simulink model "PassStCshnFldIsPosChk"  (R2018b)
settings: Solver=FixedStepDiscrete  StartTime=0.0  StopTime=10.0  RelTol=1e-3
undefined symbols (not defined in the file or in its folder): KeSMSuFirstRwStCushFoldPosDelta_Val, KeSMSuFirstRwStCushFoldPosTolr_Val
libraries: StIsPosChkLib x7, simulink x5
settings Model: Creator=sn2xws  LastModifiedBy=sn2xws
settings Model: ModifiedHistory=|
  | 2024.6.26 V3.0.0 557模式流程
  | 2024.10.14 V3.0.1 新增模式Md57，Md58
  | 25.7.1 V3.13.0 新增Md61 Md62
settings DataIOCC: SaveFormat=StructureWithTime
settings OptimizationCC: DefaultParameterBehavior=Inlined  EnhancedBackFolding=on  PassReuseOutputArgsAs=Individual arguments  ZeroExternalMemoryAtStartup=off  ZeroInternalMemoryAtStartup=off  OptimizeBlockOrder=speed  DifferentSizesBufferReuse=on  OptimizationCustomize=off
settings DebuggingCC: ParameterTunabilityLossMsg=error
settings SFSimCC: MATLABDynamicMemAlloc=off
settings RTWCC: SystemTargetFile=autosar.tlc  GenCodeOnly=on  TemplateMakefile=ert_default_tmf  Description=AUTOSAR  GenerateReport=on  IncludeHyperlinkInReport=on  LaunchReport=on  GenerateTraceInfo=on  GenerateTraceReport=on  GenerateTraceReportSl=on  GenerateTraceReportSf=on  GenerateTraceReportEml=on
settings CodeAppCC: ForceParamTrailComments=on  IgnoreCustomStorageClasses=off  OperatorAnnotations=on  SimulinkDataObjDesc=on  SFDataObjDesc=on  InsertBlockDesc=on
settings STFCustomTargetCC: TargetLangStandard=C99 (ISO)  MultiwordLength=256  ParMdlRefBuildCompliant=on  CompOptLevelCompliant=on  IncludeMdlTerminateFcn=off  CombineOutputUpdateFcns=on  SuppressErrorStatus=on  ERTCustomFileBanners=on  SupportNonFinite=off  SupportComplex=off  SupportContinuousTime=off  SupportNonInlinedSFcns=off  RemoveResetFunc=on  MATLABClassNameForMDSCustomization=Simulink.SoftwareTarget.ERTCustomization  AutosarCompliant=on  UseToolchainInfoCompliant=on  LookupTableObjectStructAxisOrder=2,1,3,4,...  LUTObjectStructOrderEvenSpacing=Size,Table,Breakpoints  SystemTargetFile=autosar.tlc
settings ERTTargetCC: TargetLangStandard=C99 (ISO)  ConcurrentExecutionCompliant=off  IncludeMdlTerminateFcn=off  SuppressErrorStatus=on  SupportNonFinite=off  SupportComplex=off  ModelStepFunctionPrototypeControlCompliant=off  CPPClassGenCompliant=off  AutosarCompliant=on  LookupTableObjectStructAxisOrder=2,1,3,4,...  LUTObjectStructOrderEvenSpacing=Size,Table,Breakpoints  InlinedParameterPlacement=NonHierarchical  ERTCustomFileTemplate=example_file_process.tlc  ERTFilePackagingFormat=Compact

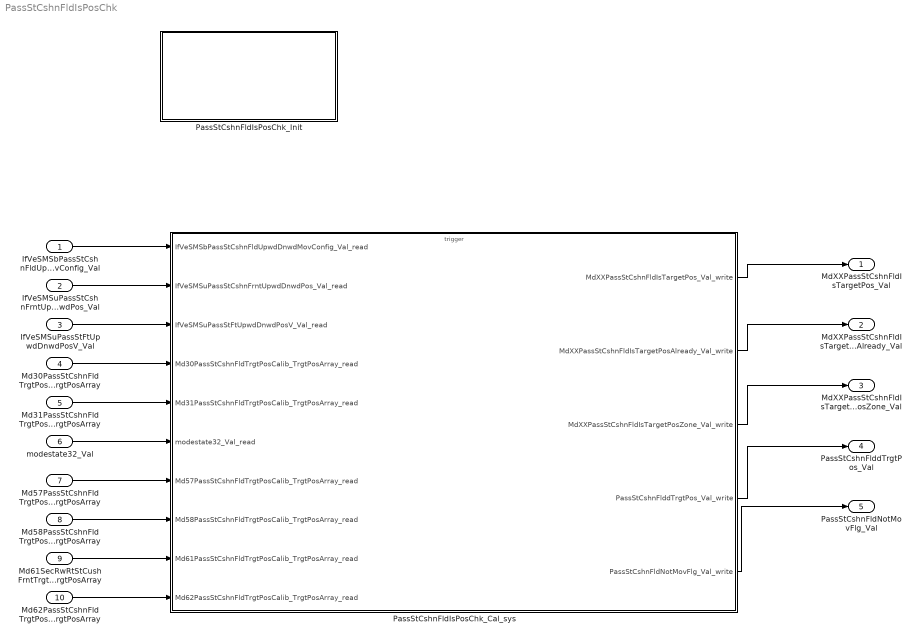
== system PassStCshnFldIsPosChk ==
  IfVeSMSbPassStCshnFldUpwdDnwdMovConfig_Val : Inport  OutDataTypeStr=boolean  PortDimensions=1
  IfVeSMSuPassStCshnFrntUpwdDnwdPos_Val : Inport  Port=2  OutDataTypeStr=uint16  PortDimensions=1
  IfVeSMSuPassStFtUpwdDnwdPosV_Val : Inport  Port=3  OutDataTypeStr=boolean  PortDimensions=1
  Md30PassStCshnFldTrgtPosCalib_TrgtPosArray : Inport  Description=|  Port=4  OutDataTypeStr=uint16  PortDimensions=3
      | 0:Pos
      | 1:Max
      | 2:Min
  Md31PassStCshnFldTrgtPosCalib_TrgtPosArray : Inport  Description=|  Port=5  OutDataTypeStr=uint16  PortDimensions=3
      | 0:Pos
      | 1:Max
      | 2:Min
  modestate32_Val : Inport  Port=6  OutDataTypeStr=uint32  PortDimensions=1
  Md57PassStCshnFldTrgtPosCalib_TrgtPosArray : Inport  Description=|  Port=7  OutDataTypeStr=uint16  PortDimensions=3
      | 0:Pos
      | 1:Max
      | 2:Min
  Md58PassStCshnFldTrgtPosCalib_TrgtPosArray : Inport  Description=|  Port=8  OutDataTypeStr=uint16  PortDimensions=3
      | 0:Pos
      | 1:Max
      | 2:Min
  Md61SecRwRtStCushFrntTrgtPosCalib_TrgtPosArray : Inport  Description=|  Port=9  OutDataTypeStr=uint16  PortDimensions=3
      | 0:Pos
      | 1:Max
      | 2:Min
  Md62PassStCshnFldTrgtPosCalib_TrgtPosArray : Inport  Description=|  Port=10  OutDataTypeStr=uint16  PortDimensions=3
      | 0:Pos
      | 1:Max
      | 2:Min
  PassStCshnFldIsPosChk_Cal_sys : Subsystem
  PassStCshnFldIsPosChk_Init : Subsystem
  MdXXPassStCshnFldIsTargetPos_Val : Outport  OutDataTypeStr=uint32  PortDimensions=1
  MdXXPassStCshnFldIsTargetPosAlready_Val : Outport  Port=2  OutDataTypeStr=uint32  PortDimensions=1
  MdXXPassStCshnFldIsTargetPosZone_Val : Outport  Port=3  OutDataTypeStr=uint32  PortDimensions=1
  PassStCshnFlddTrgtPos_Val : Outport  Port=4  OutDataTypeStr=uint16  PortDimensions=1
  PassStCshnFldNotMovFlg_Val : Outport  Port=5  OutDataTypeStr=boolean  PortDimensions=1
  wires:
  IfVeSMSbPassStCshnFldUpwdDnwdMovConfig_Val/1 -> PassStCshnFldIsPosChk_Cal_sys/1(IfVeSMSbPassStCshnFldUpwdDnwdMovConfig_Val_read)
  IfVeSMSuPassStCshnFrntUpwdDnwdPos_Val/1 -> PassStCshnFldIsPosChk_Cal_sys/2(IfVeSMSuPassStCshnFrntUpwdDnwdPos_Val_read)
  IfVeSMSuPassStFtUpwdDnwdPosV_Val/1 -> PassStCshnFldIsPosChk_Cal_sys/3(IfVeSMSuPassStFtUpwdDnwdPosV_Val_read)
  Md30PassStCshnFldTrgtPosCalib_TrgtPosArray/1 -> PassStCshnFldIsPosChk_Cal_sys/4(Md30PassStCshnFldTrgtPosCalib_TrgtPosArray_read)
  Md31PassStCshnFldTrgtPosCalib_TrgtPosArray/1 -> PassStCshnFldIsPosChk_Cal_sys/5(Md31PassStCshnFldTrgtPosCalib_TrgtPosArray_read)
  modestate32_Val/1 -> PassStCshnFldIsPosChk_Cal_sys/6(modestate32_Val_read)
  PassStCshnFldIsPosChk_Cal_sys/1(MdXXPassStCshnFldIsTargetPos_Val_write) -> MdXXPassStCshnFldIsTargetPos_Val/1
  PassStCshnFldIsPosChk_Cal_sys/2(MdXXPassStCshnFldIsTargetPosAlready_Val_write) -> MdXXPassStCshnFldIsTargetPosAlready_Val/1
  PassStCshnFldIsPosChk_Cal_sys/3(MdXXPassStCshnFldIsTargetPosZone_Val_write) -> MdXXPassStCshnFldIsTargetPosZone_Val/1
  PassStCshnFldIsPosChk_Cal_sys/4(PassStCshnFlddTrgtPos_Val_write) -> PassStCshnFlddTrgtPos_Val/1
  PassStCshnFldIsPosChk_Cal_sys/5(PassStCshnFldNotMovFlg_Val_write) -> PassStCshnFldNotMovFlg_Val/1
  Md57PassStCshnFldTrgtPosCalib_TrgtPosArray/1 -> PassStCshnFldIsPosChk_Cal_sys/7(Md57PassStCshnFldTrgtPosCalib_TrgtPosArray_read)
  Md58PassStCshnFldTrgtPosCalib_TrgtPosArray/1 -> PassStCshnFldIsPosChk_Cal_sys/8(Md58PassStCshnFldTrgtPosCalib_TrgtPosArray_read)
  Md61SecRwRtStCushFrntTrgtPosCalib_TrgtPosArray/1 -> PassStCshnFldIsPosChk_Cal_sys/9(Md61PassStCshnFldTrgtPosCalib_TrgtPosArray_read)
  Md62PassStCshnFldTrgtPosCalib_TrgtPosArray/1 -> PassStCshnFldIsPosChk_Cal_sys/10(Md62PassStCshnFldTrgtPosCalib_TrgtPosArray_read)

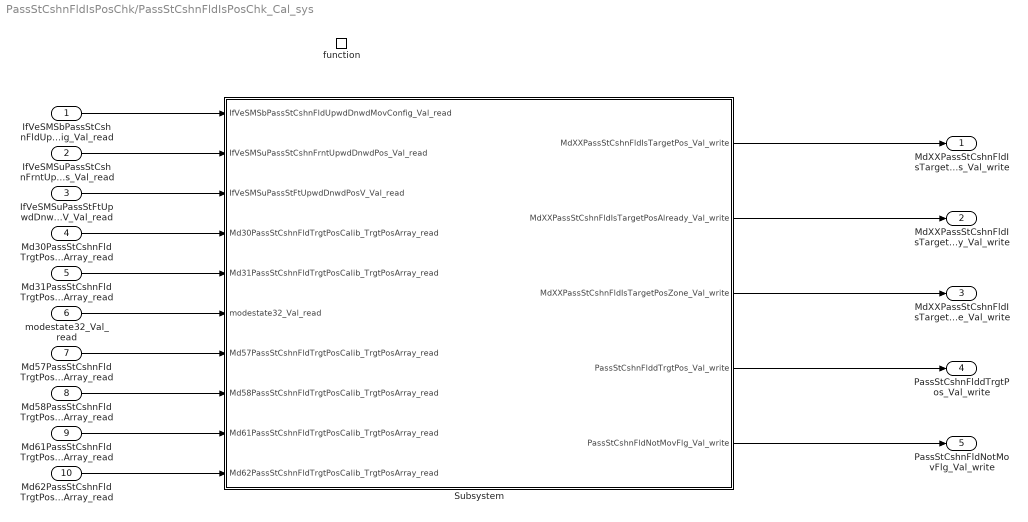
== system PassStCshnFldIsPosChk/PassStCshnFldIsPosChk_Cal_sys ==
  IfVeSMSbPassStCshnFldUpwdDnwdMovConfig_Val_read : Inport
  IfVeSMSuPassStCshnFrntUpwdDnwdPos_Val_read : Inport  Port=2
  IfVeSMSuPassStFtUpwdDnwdPosV_Val_read : Inport  Port=3
  Md30PassStCshnFldTrgtPosCalib_TrgtPosArray_read : Inport  Port=4
  Md31PassStCshnFldTrgtPosCalib_TrgtPosArray_read : Inport  Port=5
  modestate32_Val_read : Inport  Port=6
  Md57PassStCshnFldTrgtPosCalib_TrgtPosArray_read : Inport  Port=7
  Md58PassStCshnFldTrgtPosCalib_TrgtPosArray_read : Inport  Port=8
  Md61PassStCshnFldTrgtPosCalib_TrgtPosArray_read : Inport  Port=9
  Md62PassStCshnFldTrgtPosCalib_TrgtPosArray_read : Inport  Port=10
  function : TriggerPort  TriggerType=function-call  IsSimulinkFunction=on  FunctionName=PassStCshnFldIsPosChk_Cal  VariantControl=(inherit)
  Subsystem : Subsystem
  MdXXPassStCshnFldIsTargetPos_Val_write : Outport
      settings: EnsureOutportIsVirtual=on
  MdXXPassStCshnFldIsTargetPosAlready_Val_write : Outport  Port=2
      settings: EnsureOutportIsVirtual=on
  MdXXPassStCshnFldIsTargetPosZone_Val_write : Outport  Port=3
      settings: EnsureOutportIsVirtual=on
  PassStCshnFlddTrgtPos_Val_write : Outport  Port=4
      settings: EnsureOutportIsVirtual=on
  PassStCshnFldNotMovFlg_Val_write : Outport  Port=5
      settings: EnsureOutportIsVirtual=on
  wires:
  IfVeSMSbPassStCshnFldUpwdDnwdMovConfig_Val_read/1 -> Subsystem/1(IfVeSMSbPassStCshnFldUpwdDnwdMovConfig_Val_read)
  IfVeSMSuPassStCshnFrntUpwdDnwdPos_Val_read/1 -> Subsystem/2(IfVeSMSuPassStCshnFrntUpwdDnwdPos_Val_read)
  IfVeSMSuPassStFtUpwdDnwdPosV_Val_read/1 -> Subsystem/3(IfVeSMSuPassStFtUpwdDnwdPosV_Val_read)
  Md30PassStCshnFldTrgtPosCalib_TrgtPosArray_read/1 -> Subsystem/4(Md30PassStCshnFldTrgtPosCalib_TrgtPosArray_read)
  Md31PassStCshnFldTrgtPosCalib_TrgtPosArray_read/1 -> Subsystem/5(Md31PassStCshnFldTrgtPosCalib_TrgtPosArray_read)
  modestate32_Val_read/1 -> Subsystem/6(modestate32_Val_read)
  Subsystem/1(MdXXPassStCshnFldIsTargetPos_Val_write) -> MdXXPassStCshnFldIsTargetPos_Val_write/1
  Subsystem/2(MdXXPassStCshnFldIsTargetPosAlready_Val_write) -> MdXXPassStCshnFldIsTargetPosAlready_Val_write/1
  Subsystem/3(MdXXPassStCshnFldIsTargetPosZone_Val_write) -> MdXXPassStCshnFldIsTargetPosZone_Val_write/1
  Subsystem/4(PassStCshnFlddTrgtPos_Val_write) -> PassStCshnFlddTrgtPos_Val_write/1
  Subsystem/5(PassStCshnFldNotMovFlg_Val_write) -> PassStCshnFldNotMovFlg_Val_write/1
  Md57PassStCshnFldTrgtPosCalib_TrgtPosArray_read/1 -> Subsystem/7(Md57PassStCshnFldTrgtPosCalib_TrgtPosArray_read)
  Md58PassStCshnFldTrgtPosCalib_TrgtPosArray_read/1 -> Subsystem/8(Md58PassStCshnFldTrgtPosCalib_TrgtPosArray_read)
  Md61PassStCshnFldTrgtPosCalib_TrgtPosArray_read/1 -> Subsystem/9(Md61PassStCshnFldTrgtPosCalib_TrgtPosArray_read)
  Md62PassStCshnFldTrgtPosCalib_TrgtPosArray_read/1 -> Subsystem/10(Md62PassStCshnFldTrgtPosCalib_TrgtPosArray_read)

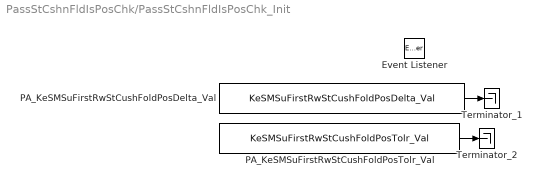
== system PassStCshnFldIsPosChk/PassStCshnFldIsPosChk_Init ==
  Event Listener : EventListener  EventName=reset
  PA_KeSMSuFirstRwStCushFoldPosDelta_Val : Constant  Value=KeSMSuFirstRwStCushFoldPosDelta_Val
  PA_KeSMSuFirstRwStCushFoldPosTolr_Val : Constant  Value=KeSMSuFirstRwStCushFoldPosTolr_Val
  Terminator_1 : Terminator
  Terminator_2 : Terminator
  wires:
  PA_KeSMSuFirstRwStCushFoldPosDelta_Val/1 -> Terminator_1/1
  PA_KeSMSuFirstRwStCushFoldPosTolr_Val/1 -> Terminator_2/1

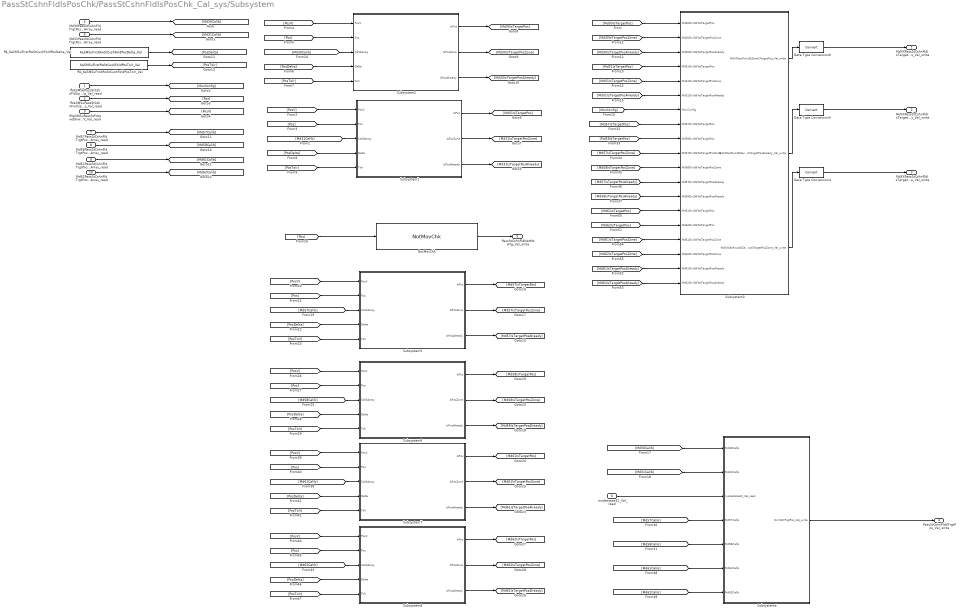
== system PassStCshnFldIsPosChk/PassStCshnFldIsPosChk_Cal_sys/Subsystem ==
  IfVeSMSbPassStCshnFldUpwdDnwdMovConfig_Val_read : Inport
  IfVeSMSuPassStCshnFrntUpwdDnwdPos_Val_read : Inport  Port=2
  IfVeSMSuPassStFtUpwdDnwdPosV_Val_read : Inport  Port=3
  Md30PassStCshnFldTrgtPosCalib_TrgtPosArray_read : Inport  Port=4
  Md31PassStCshnFldTrgtPosCalib_TrgtPosArray_read : Inport  Port=5
  modestate32_Val_read : Inport  Port=6
  Md57PassStCshnFldTrgtPosCalib_TrgtPosArray_read : Inport  Port=7
  Md58PassStCshnFldTrgtPosCalib_TrgtPosArray_read : Inport  Port=8
  Md61PassStCshnFldTrgtPosCalib_TrgtPosArray_read : Inport  Port=9
  Md62PassStCshnFldTrgtPosCalib_TrgtPosArray_read : Inport  Port=10
  Data Type Conversion4 : DataTypeConversion
  Data Type Conversion5 : DataTypeConversion
  Data Type Conversion6 : DataTypeConversion
  NotMovChk : StIsPosChkLib/NotMovChk  SystemSampleTime=-1
  PA_KeSMSuFirstRwStCushFoldPosDelta_Val : Constant  Value=KeSMSuFirstRwStCushFoldPosDelta_Val
  PA_KeSMSuFirstRwStCushFoldPosTolr_Val : Constant  Value=KeSMSuFirstRwStCushFoldPosTolr_Val
  Subsystem1 : Subsystem
  Subsystem2 : Subsystem
  Subsystem3 : Subsystem
  Subsystem4 : Subsystem
  Subsystem5 : Subsystem
  Subsystem6 : Subsystem
  Subsystem7 : Subsystem
  Subsystem8 : Subsystem
  MdXXPassStCshnFldIsTargetPos_Val_write : Outport
      settings: EnsureOutportIsVirtual=on
  MdXXPassStCshnFldIsTargetPosAlready_Val_write : Outport  Port=2
      settings: EnsureOutportIsVirtual=on
  MdXXPassStCshnFldIsTargetPosZone_Val_write : Outport  Port=3
      settings: EnsureOutportIsVirtual=on
  PassStCshnFlddTrgtPos_Val_write : Outport  Port=4
      settings: EnsureOutportIsVirtual=on
  PassStCshnFldNotMovFlg_Val_write : Outport  Port=5
      settings: EnsureOutportIsVirtual=on
  wires:
  modestate32_Val_read/1 -> Subsystem4/3(modestate32_Val_read)
  PA_KeSMSuFirstRwStCushFoldPosDelta_Val/1 -> [PosDelta]
  Md30PassStCshnFldTrgtPosCalib_TrgtPosArray_read/1 -> [Md30Calib]
  Md31PassStCshnFldTrgtPosCalib_TrgtPosArray_read/1 -> [Md31Calib]
  IfVeSMSbPassStCshnFldUpwdDnwdMovConfig_Val_read/1 -> [MovConfig]
  IfVeSMSuPassStCshnFrntUpwdDnwdPos_Val_read/1 -> [Pos]
  IfVeSMSuPassStFtUpwdDnwdPosV_Val_read/1 -> [PosV]
  PA_KeSMSuFirstRwStCushFoldPosTolr_Val/1 -> [PosTolr]
  Data Type Conversion4/1 -> MdXXPassStCshnFldIsTargetPosZone_Val_write/1
  Data Type Conversion6/1 -> MdXXPassStCshnFldIsTargetPos_Val_write/1
  Subsystem3/3(MdXXSecRwLtStZeroIsTargetPosZone_Val_write) -> Data Type Conversion4/1
  Subsystem3/2(MdXXSecRwLtStZeroIsTargetPosAlready_Val_write) -> Data Type Conversion5/1
  [MovConfig] -> Subsystem3/7(MovConfig)
  [Md30IsTargetPosAlready] -> Subsystem3/3(Md30DrvStFtIsTargetPosAlready)
  Data Type Conversion5/1 -> MdXXPassStCshnFldIsTargetPosAlready_Val_write/1
  [PosTolr] -> Subsystem1/5(Tolr)
  [Md31Calib] -> Subsystem1/3(CalibArray)
  Subsystem1/3(IsPosAlready) -> [Md31IsTargetPosAlready]
  [PosDelta] -> Subsystem1/4(Delta)
  [Pos] -> Subsystem1/2(Pos)
  [PosV] -> Subsystem1/1(PosV)
  Subsystem1/1(IsPos) -> [Md31IsTargetPos]
  Subsystem1/2(IsPosZone) -> [Md31IsTargetPosZone]
  [PosTolr] -> Subsystem2/5(Tolr)
  [PosV] -> Subsystem2/1(PosV)
  Subsystem2/2(IsPosZone) -> [Md30IsTargetPosZone]
  [Md30IsTargetPos] -> Subsystem3/1(Md30DrvStFtIsTargetPos)
  [Md31IsTargetPosZone] -> Subsystem3/5(Md31DrvStFtIsTargetPosZone)
  Subsystem2/1(IsPos) -> [Md30IsTargetPos]
  [Pos] -> Subsystem2/2(Pos)
  [Md31IsTargetPosAlready] -> Subsystem3/6(Md31DrvStFtIsTargetPosAlready)
  [PosDelta] -> Subsystem2/4(Delta)
  [Md30Calib] -> Subsystem2/3(CalibArray)
  Subsystem3/1(MdXXSecRwLtStZeroIsTargetPos_Val_write) -> Data Type Conversion6/1
  Subsystem2/3(IsPosAlready) -> [Md30IsTargetPosAlready]
  [Md31IsTargetPos] -> Subsystem3/4(Md31DrvStFtIsTargetPos)
  [Md30IsTargetPosZone] -> Subsystem3/2(Md30DrvStFtIsTargetPosZone)
  NotMovChk/1 -> PassStCshnFldNotMovFlg_Val_write/1
  [Pos] -> NotMovChk/1
  [Md31Calib] -> Subsystem4/2(Md31Calib)
  Subsystem4/1(DrvStFtTrgtPos_Val_write) -> PassStCshnFlddTrgtPos_Val_write/1
  [Md30Calib] -> Subsystem4/1(Md30Calib)
  Md57PassStCshnFldTrgtPosCalib_TrgtPosArray_read/1 -> [Md57Calib]
  Md58PassStCshnFldTrgtPosCalib_TrgtPosArray_read/1 -> [Md58Calib]
  Subsystem5/2(IsPosZone) -> [Md57IsTargetPosZone]
  Subsystem5/1(IsPos) -> [Md57IsTargetPos]
  [PosV] -> Subsystem5/1(PosV)
  [Pos] -> Subsystem5/2(Pos)
  [PosDelta] -> Subsystem5/4(Delta)
  Subsystem5/3(IsPosAlready) -> [Md57IsTargetPosAlready]
  [Md57Calib] -> Subsystem5/3(CalibArray)
  [PosTolr] -> Subsystem5/5(Tolr)
  [PosTolr] -> Subsystem6/5(Tolr)
  [Md58Calib] -> Subsystem6/3(CalibArray)
  Subsystem6/3(IsPosAlready) -> [Md58IsTargetPosAlready]
  [PosDelta] -> Subsystem6/4(Delta)
  [Pos] -> Subsystem6/2(Pos)
  [PosV] -> Subsystem6/1(PosV)
  Subsystem6/1(IsPos) -> [Md58IsTargetPos]
  Subsystem6/2(IsPosZone) -> [Md58IsTargetPosZone]
  [Md57Calib] -> Subsystem4/4(Md57Calib)
  [Md58Calib] -> Subsystem4/5(Md58Calib)
  [Md57IsTargetPos] -> Subsystem3/8(Md57DrvStFtIsTargetPos)
  [Md58IsTargetPos] -> Subsystem3/9(Md58DrvStFtIsTargetPos)
  [Md57IsTargetPosZone] -> Subsystem3/10(Md57DrvStFtIsTargetPosZone)
  [Md58IsTargetPosZone] -> Subsystem3/11(Md58DrvStFtIsTargetPosZone)
  [Md58IsTargetPosAlready] -> Subsystem3/13(Md58DrvStFtIsTargetPosAlready)
  [Md57IsTargetPosAlready] -> Subsystem3/12(Md57DrvStFtIsTargetPosAlready)
  Md61PassStCshnFldTrgtPosCalib_TrgtPosArray_read/1 -> [Md61Calib]
  Md62PassStCshnFldTrgtPosCalib_TrgtPosArray_read/1 -> [Md62Calib]
  Subsystem7/2(IsPosZone) -> [Md61IsTargetPosZone]
  Subsystem7/1(IsPos) -> [Md61IsTargetPos]
  [PosV] -> Subsystem7/1(PosV)
  [Pos] -> Subsystem7/2(Pos)
  [PosDelta] -> Subsystem7/4(Delta)
  Subsystem7/3(IsPosAlready) -> [Md61IsTargetPosAlready]
  [Md61Calib] -> Subsystem7/3(CalibArray)
  [PosTolr] -> Subsystem7/5(Tolr)
  [PosTolr] -> Subsystem8/5(Tolr)
  [Md62Calib] -> Subsystem8/3(CalibArray)
  Subsystem8/3(IsPosAlready) -> [Md62IsTargetPosAlready]
  [PosDelta] -> Subsystem8/4(Delta)
  [Pos] -> Subsystem8/2(Pos)
  [PosV] -> Subsystem8/1(PosV)
  Subsystem8/1(IsPos) -> [Md62IsTargetPos]
  Subsystem8/2(IsPosZone) -> [Md62IsTargetPosZone]
  [Md61Calib] -> Subsystem4/6(Md61Calib)
  [Md62Calib] -> Subsystem4/7(Md62Calib)
  [Md61IsTargetPos] -> Subsystem3/14(Md61DrvStFtIsTargetPos)
  [Md62IsTargetPos] -> Subsystem3/15(Md62DrvStFtIsTargetPos)
  [Md61IsTargetPosZone] -> Subsystem3/16(Md61DrvStFtIsTargetPosZone)
  [Md62IsTargetPosZone] -> Subsystem3/17(Md62DrvStFtIsTargetPosZone)
  [Md61IsTargetPosAlready] -> Subsystem3/18(Md61DrvStFtIsTargetPosAlready)
  [Md62IsTargetPosAlready] -> Subsystem3/19(Md62DrvStFtIsTargetPosAlready)

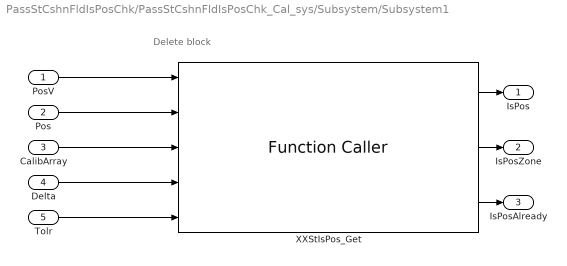
== system PassStCshnFldIsPosChk/PassStCshnFldIsPosChk_Cal_sys/Subsystem/Subsystem1 ==
  note: Delete block
  PosV : Inport
  Pos : Inport  Port=2
  CalibArray : Inport  Port=3
  Delta : Inport  Port=4
  Tolr : Inport  Port=5
  XXStIsPos_Get : FunctionCaller  FunctionPrototype=[IsPos,IsPosZone,IsPosAlready] = XXStIsPos_Get(PosV,Pos,CalibArray,Delta,Tolr)  InputArgumentSpecifications=boolean(true), uint16(1), uint16([1;1;1]), uint16(1), uint16(1)  OutputArgumentSpecifications=boolean(true), boolean(true), boolean(true)
  IsPos : Outport
  IsPosZone : Outport  Port=2
  IsPosAlready : Outport  Port=3
  wires:
  Delta/1 -> XXStIsPos_Get/4
  Tolr/1 -> XXStIsPos_Get/5
  PosV/1 -> XXStIsPos_Get/1
  XXStIsPos_Get/2 -> IsPosZone/1
  Pos/1 -> XXStIsPos_Get/2
  XXStIsPos_Get/1 -> IsPos/1
  CalibArray/1 -> XXStIsPos_Get/3
  XXStIsPos_Get/3 -> IsPosAlready/1

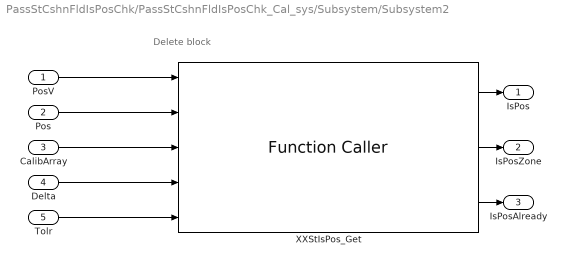
== system PassStCshnFldIsPosChk/PassStCshnFldIsPosChk_Cal_sys/Subsystem/Subsystem2 ==
  note: Delete block
  PosV : Inport
  Pos : Inport  Port=2
  CalibArray : Inport  Port=3
  Delta : Inport  Port=4
  Tolr : Inport  Port=5
  XXStIsPos_Get : FunctionCaller  FunctionPrototype=[IsPos,IsPosZone,IsPosAlready] = XXStIsPos_Get(PosV,Pos,CalibArray,Delta,Tolr)  InputArgumentSpecifications=boolean(true), uint16(1), uint16([1;1;1]), uint16(1), uint16(1)  OutputArgumentSpecifications=boolean(true), boolean(true), boolean(true)
  IsPos : Outport
  IsPosZone : Outport  Port=2
  IsPosAlready : Outport  Port=3
  wires:
  XXStIsPos_Get/3 -> IsPosAlready/1
  CalibArray/1 -> XXStIsPos_Get/3
  XXStIsPos_Get/1 -> IsPos/1
  Pos/1 -> XXStIsPos_Get/2
  XXStIsPos_Get/2 -> IsPosZone/1
  PosV/1 -> XXStIsPos_Get/1
  Tolr/1 -> XXStIsPos_Get/5
  Delta/1 -> XXStIsPos_Get/4

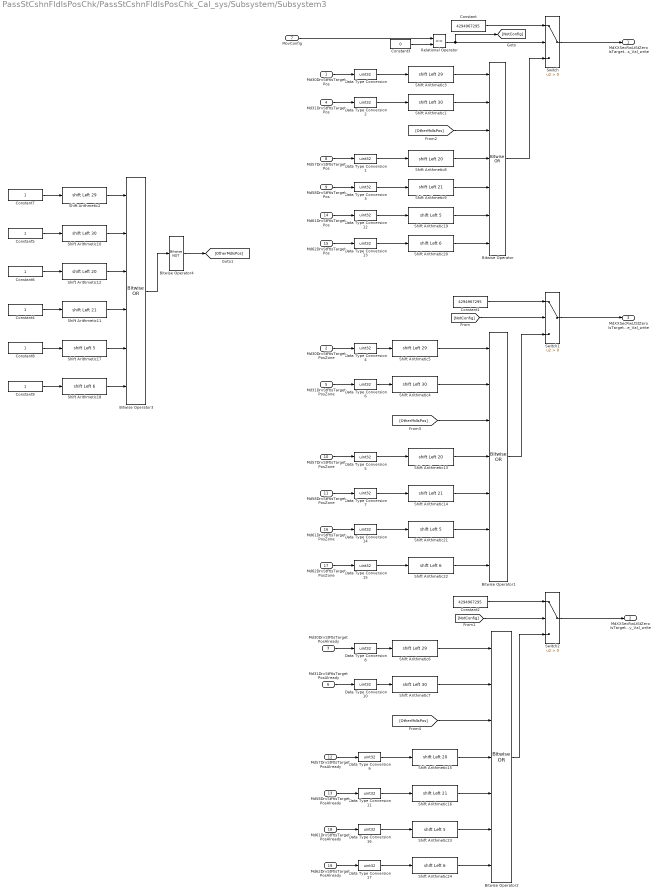
== system PassStCshnFldIsPosChk/PassStCshnFldIsPosChk_Cal_sys/Subsystem/Subsystem3 ==
  Md30DrvStFtIsTargetPos : Inport
  Md30DrvStFtIsTargetPosZone : Inport  Port=2
  Md30DrvStFtIsTargetPosAlready : Inport  Port=3
  Md31DrvStFtIsTargetPos : Inport  Port=4
  Md31DrvStFtIsTargetPosZone : Inport  Port=5
  Md31DrvStFtIsTargetPosAlready : Inport  Port=6
  MovConfig : Inport  Port=7
  Md57DrvStFtIsTargetPos : Inport  Port=8
  Md58DrvStFtIsTargetPos : Inport  Port=9
  Md57DrvStFtIsTargetPosZone : Inport  Port=10
  Md58DrvStFtIsTargetPosZone : Inport  Port=11
  Md57DrvStFtIsTargetPosAlready : Inport  Port=12
  Md58DrvStFtIsTargetPosAlready : Inport  Port=13
  Md61DrvStFtIsTargetPos : Inport  Port=14
  Md62DrvStFtIsTargetPos : Inport  Port=15
  Md61DrvStFtIsTargetPosZone : Inport  Port=16
  Md62DrvStFtIsTargetPosZone : Inport  Port=17
  Md61DrvStFtIsTargetPosAlready : Inport  Port=18
  Md62DrvStFtIsTargetPosAlready : Inport  Port=19
  Bitwise Operator : simulink/Logic and Bit Operations/Bitwise Operator  logicop=OR  UseBitMask=off  NumInputPorts=7  BitMask=bin2dec('11011001')  BitMaskRealWorld=Stored Integer
  Bitwise Operator1 : simulink/Logic and Bit Operations/Bitwise Operator  logicop=OR  UseBitMask=off  NumInputPorts=7  BitMask=bin2dec('11011001')  BitMaskRealWorld=Stored Integer
  Bitwise Operator2 : simulink/Logic and Bit Operations/Bitwise Operator  logicop=OR  UseBitMask=off  NumInputPorts=7  BitMask=bin2dec('11011001')  BitMaskRealWorld=Stored Integer
  Bitwise Operator3 : simulink/Logic and Bit Operations/Bitwise Operator  logicop=OR  UseBitMask=off  NumInputPorts=6  BitMask=bin2dec('11011001')  BitMaskRealWorld=Stored Integer
  Bitwise Operator4 : simulink/Logic and Bit Operations/Bitwise Operator  logicop=NOT  UseBitMask=off  BitMask=bin2dec('11011001')  BitMaskRealWorld=Stored Integer
  Constant : Constant  Value=4294967295  OutDataTypeStr=uint32
  Constant1 : Constant  Value=4294967295  OutDataTypeStr=uint32
  Constant2 : Constant  Value=4294967295  OutDataTypeStr=uint32
  Constant3 : Constant  Value=0  OutDataTypeStr=uint8
  Constant{4..9} (6 alike) : Constant  OutDataTypeStr=uint32
  Data Type Conversion{,1..17} (18 alike) : DataTypeConversion  OutDataTypeStr=uint32
  Relational Operator : RelationalOperator  Operator===  OutDataTypeStr=boolean  RndMeth=Simplest
  Shift Arithmetic{1,4,7,10} (4 alike) : ArithShift  BitShiftNumber=30  BitShiftDirection=Left
  Shift Arithmetic{9,11,14,16} (4 alike) : ArithShift  BitShiftNumber=21  BitShiftDirection=Left
  Shift Arithmetic{8,12..13,15} (4 alike) : ArithShift  BitShiftNumber=20  BitShiftDirection=Left
  Shift Arithmetic{17,19,21,23} (4 alike) : ArithShift  BitShiftNumber=5  BitShiftDirection=Left
  Shift Arithmetic{18,20,22,24} (4 alike) : ArithShift  BitShiftNumber=6  BitShiftDirection=Left
  Shift Arithmetic{2..3,5..6} (4 alike) : ArithShift  BitShiftNumber=29  BitShiftDirection=Left
  Switch : Switch  Criteria=u2 > Threshold
  Switch1 : Switch  Criteria=u2 > Threshold
  Switch2 : Switch  Criteria=u2 > Threshold
  MdXXSecRwLtStZeroIsTargetPos_Val_write : Outport
      settings: EnsureOutportIsVirtual=on
  MdXXSecRwLtStZeroIsTargetPosAlready_Val_write : Outport  Port=2
      settings: EnsureOutportIsVirtual=on
  MdXXSecRwLtStZeroIsTargetPosZone_Val_write : Outport  Port=3
      settings: EnsureOutportIsVirtual=on
  wires:
  Switch/1 -> MdXXSecRwLtStZeroIsTargetPos_Val_write/1
  Relational Operator/1 -> [NotConfig], Switch/2
  Constant/1 -> Switch/1
  [NotConfig] -> Switch1/2
  MovConfig/1 -> Relational Operator/1
  Constant1/1 -> Switch1/1
  Constant2/1 -> Switch2/1
  [NotConfig] -> Switch2/2
  Md30DrvStFtIsTargetPos/1 -> Data Type Conversion/1
  Md31DrvStFtIsTargetPos/1 -> Data Type Conversion2/1
  Shift Arithmetic1/1 -> Bitwise Operator/2
  Bitwise Operator1/1 -> Switch1/3
  Bitwise Operator2/1 -> Switch2/3
  Data Type Conversion2/1 -> Shift Arithmetic1/1
  Data Type Conversion6/1 -> Shift Arithmetic4/1
  Data Type Conversion4/1 -> Shift Arithmetic5/1
  Shift Arithmetic4/1 -> Bitwise Operator1/2
  Md31DrvStFtIsTargetPosZone/1 -> Data Type Conversion6/1
  Md30DrvStFtIsTargetPosZone/1 -> Data Type Conversion4/1
  Shift Arithmetic7/1 -> Bitwise Operator2/2
  Data Type Conversion8/1 -> Shift Arithmetic6/1
  Data Type Conversion10/1 -> Shift Arithmetic7/1
  Md30DrvStFtIsTargetPosAlready/1 -> Data Type Conversion8/1
  Md31DrvStFtIsTargetPosAlready/1 -> Data Type Conversion10/1
  Data Type Conversion/1 -> Shift Arithmetic3/1
  Bitwise Operator/1 -> Switch/3
  Switch2/1 -> MdXXSecRwLtStZeroIsTargetPosAlready_Val_write/1
  Switch1/1 -> MdXXSecRwLtStZeroIsTargetPosZone_Val_write/1
  Constant3/1 -> Relational Operator/2
  Constant5/1 -> Shift Arithmetic10/1
  Shift Arithmetic10/1 -> Bitwise Operator3/2
  Constant7/1 -> Shift Arithmetic2/1
  Bitwise Operator3/1 -> Bitwise Operator4/1
  Bitwise Operator4/1 -> [OtherMdIsPos]
  [OtherMdIsPos] -> Bitwise Operator/3
  [OtherMdIsPos] -> Bitwise Operator1/3
  [OtherMdIsPos] -> Bitwise Operator2/3
  Shift Arithmetic2/1 -> Bitwise Operator3/1
  Shift Arithmetic3/1 -> Bitwise Operator/1
  Shift Arithmetic5/1 -> Bitwise Operator1/1
  Shift Arithmetic6/1 -> Bitwise Operator2/1
  Md57DrvStFtIsTargetPos/1 -> Data Type Conversion1/1
  Md58DrvStFtIsTargetPos/1 -> Data Type Conversion3/1
  Data Type Conversion1/1 -> Shift Arithmetic8/1
  Data Type Conversion3/1 -> Shift Arithmetic9/1
  Shift Arithmetic8/1 -> Bitwise Operator/4
  Shift Arithmetic9/1 -> Bitwise Operator/5
  Shift Arithmetic12/1 -> Bitwise Operator3/3
  Constant6/1 -> Shift Arithmetic12/1
  Shift Arithmetic11/1 -> Bitwise Operator3/4
  Constant4/1 -> Shift Arithmetic11/1
  Shift Arithmetic14/1 -> Bitwise Operator1/5
  Shift Arithmetic13/1 -> Bitwise Operator1/4
  Data Type Conversion7/1 -> Shift Arithmetic14/1
  Data Type Conversion5/1 -> Shift Arithmetic13/1
  Md58DrvStFtIsTargetPosZone/1 -> Data Type Conversion7/1
  Md57DrvStFtIsTargetPosZone/1 -> Data Type Conversion5/1
  Md57DrvStFtIsTargetPosAlready/1 -> Data Type Conversion9/1
  Md58DrvStFtIsTargetPosAlready/1 -> Data Type Conversion11/1
  Data Type Conversion9/1 -> Shift Arithmetic15/1
  Data Type Conversion11/1 -> Shift Arithmetic16/1
  Shift Arithmetic15/1 -> Bitwise Operator2/4
  Shift Arithmetic16/1 -> Bitwise Operator2/5
  Constant8/1 -> Shift Arithmetic17/1
  Shift Arithmetic17/1 -> Bitwise Operator3/5
  Shift Arithmetic18/1 -> Bitwise Operator3/6
  Constant9/1 -> Shift Arithmetic18/1
  Shift Arithmetic19/1 -> Bitwise Operator/6
  Data Type Conversion12/1 -> Shift Arithmetic19/1
  Md61DrvStFtIsTargetPos/1 -> Data Type Conversion12/1
  Md62DrvStFtIsTargetPos/1 -> Data Type Conversion13/1
  Data Type Conversion13/1 -> Shift Arithmetic20/1
  Shift Arithmetic20/1 -> Bitwise Operator/7
  Md61DrvStFtIsTargetPosZone/1 -> Data Type Conversion14/1
  Data Type Conversion14/1 -> Shift Arithmetic21/1
  Shift Arithmetic21/1 -> Bitwise Operator1/6
  Shift Arithmetic22/1 -> Bitwise Operator1/7
  Data Type Conversion15/1 -> Shift Arithmetic22/1
  Md62DrvStFtIsTargetPosZone/1 -> Data Type Conversion15/1
  Shift Arithmetic23/1 -> Bitwise Operator2/6
  Data Type Conversion16/1 -> Shift Arithmetic23/1
  Md61DrvStFtIsTargetPosAlready/1 -> Data Type Conversion16/1
  Md62DrvStFtIsTargetPosAlready/1 -> Data Type Conversion17/1
  Data Type Conversion17/1 -> Shift Arithmetic24/1
  Shift Arithmetic24/1 -> Bitwise Operator2/7

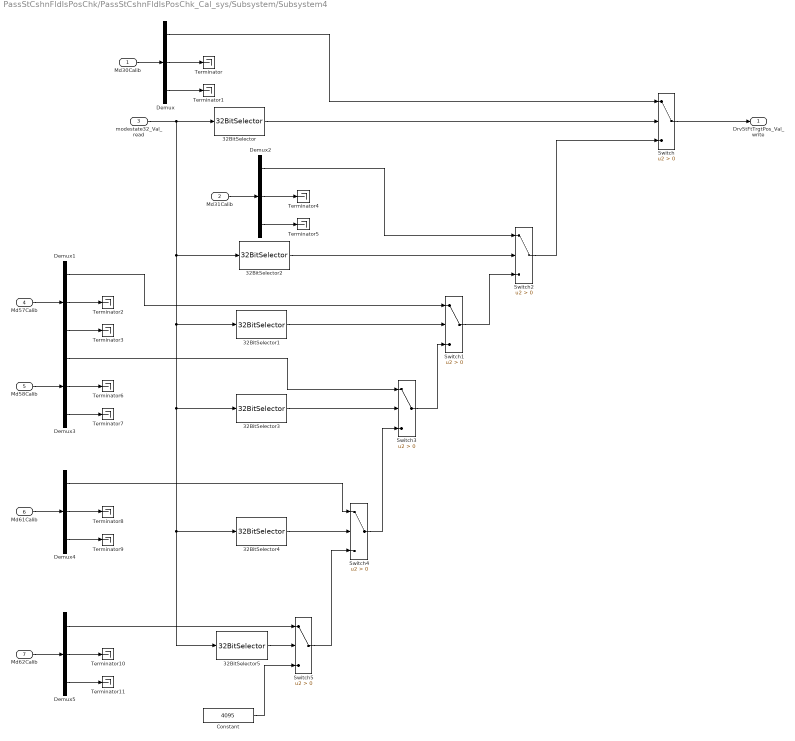
== system PassStCshnFldIsPosChk/PassStCshnFldIsPosChk_Cal_sys/Subsystem/Subsystem4 ==
  Md30Calib : Inport
  Md31Calib : Inport  Port=2
  modestate32_Val_read : Inport  Port=3
  Md57Calib : Inport  Port=4
  Md58Calib : Inport  Port=5
  Md61Calib : Inport  Port=6
  Md62Calib : Inport  Port=7
  32BitSelector : StIsPosChkLib/32BitSelector  BitNum=29
  32BitSelector1 : StIsPosChkLib/32BitSelector  BitNum=20
  32BitSelector2 : StIsPosChkLib/32BitSelector  BitNum=30
  32BitSelector3 : StIsPosChkLib/32BitSelector  BitNum=21
  32BitSelector4 : StIsPosChkLib/32BitSelector  BitNum=5
  32BitSelector5 : StIsPosChkLib/32BitSelector  BitNum=6
  Constant : Constant  Value=4095  OutDataTypeStr=uint16
  Demux{,1..5} (6 alike) : Demux  Outputs=3
  Switch{,1..5} (6 alike) : Switch  Criteria=u2 > Threshold
  Terminator{,1..11} (12 alike) : Terminator
  DrvStFtTrgtPos_Val_write : Outport
      settings: EnsureOutportIsVirtual=on
  wires:
  Md30Calib/1 -> Demux/1
  Demux/3 -> Terminator1/1
  Demux/2 -> Terminator/1
  Demux2/3 -> Terminator5/1
  Demux2/2 -> Terminator4/1
  Md31Calib/1 -> Demux2/1
  modestate32_Val_read/1 -> 32BitSelector1/1, 32BitSelector5/1, 32BitSelector4/1, 32BitSelector3/1, 32BitSelector2/1, 32BitSelector/1
  32BitSelector/1 -> Switch/2
  Demux/1 -> Switch/1
  Switch/1 -> DrvStFtTrgtPos_Val_write/1
  32BitSelector2/1 -> Switch2/2
  Demux2/1 -> Switch2/1
  Switch2/1 -> Switch/3
  Switch1/1 -> Switch2/3
  Switch3/1 -> Switch1/3
  32BitSelector1/1 -> Switch1/2
  32BitSelector3/1 -> Switch3/2
  Demux1/1 -> Switch1/1
  Md57Calib/1 -> Demux1/1
  Demux1/2 -> Terminator2/1
  Demux1/3 -> Terminator3/1
  Demux3/3 -> Terminator7/1
  Demux3/2 -> Terminator6/1
  Md58Calib/1 -> Demux3/1
  Demux3/1 -> Switch3/1
  Switch4/1 -> Switch3/3
  Switch5/1 -> Switch4/3
  32BitSelector4/1 -> Switch4/2
  32BitSelector5/1 -> Switch5/2
  Constant/1 -> Switch5/3
  Demux4/1 -> Switch4/1
  Md61Calib/1 -> Demux4/1
  Demux4/2 -> Terminator8/1
  Demux4/3 -> Terminator9/1
  Demux5/3 -> Terminator11/1
  Demux5/2 -> Terminator10/1
  Md62Calib/1 -> Demux5/1
  Demux5/1 -> Switch5/1

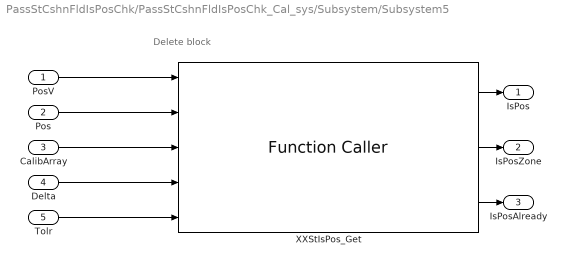
== system PassStCshnFldIsPosChk/PassStCshnFldIsPosChk_Cal_sys/Subsystem/Subsystem5 ==
  note: Delete block
  PosV : Inport
  Pos : Inport  Port=2
  CalibArray : Inport  Port=3
  Delta : Inport  Port=4
  Tolr : Inport  Port=5
  XXStIsPos_Get : FunctionCaller  FunctionPrototype=[IsPos,IsPosZone,IsPosAlready] = XXStIsPos_Get(PosV,Pos,CalibArray,Delta,Tolr)  InputArgumentSpecifications=boolean(true), uint16(1), uint16([1;1;1]), uint16(1), uint16(1)  OutputArgumentSpecifications=boolean(true), boolean(true), boolean(true)
  IsPos : Outport
  IsPosZone : Outport  Port=2
  IsPosAlready : Outport  Port=3
  wires:
  XXStIsPos_Get/3 -> IsPosAlready/1
  CalibArray/1 -> XXStIsPos_Get/3
  XXStIsPos_Get/1 -> IsPos/1
  Pos/1 -> XXStIsPos_Get/2
  XXStIsPos_Get/2 -> IsPosZone/1
  PosV/1 -> XXStIsPos_Get/1
  Tolr/1 -> XXStIsPos_Get/5
  Delta/1 -> XXStIsPos_Get/4

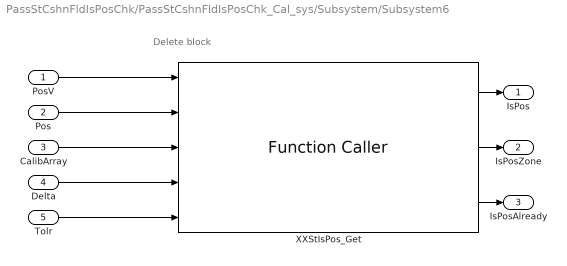
== system PassStCshnFldIsPosChk/PassStCshnFldIsPosChk_Cal_sys/Subsystem/Subsystem6 ==
  note: Delete block
  PosV : Inport
  Pos : Inport  Port=2
  CalibArray : Inport  Port=3
  Delta : Inport  Port=4
  Tolr : Inport  Port=5
  XXStIsPos_Get : FunctionCaller  FunctionPrototype=[IsPos,IsPosZone,IsPosAlready] = XXStIsPos_Get(PosV,Pos,CalibArray,Delta,Tolr)  InputArgumentSpecifications=boolean(true), uint16(1), uint16([1;1;1]), uint16(1), uint16(1)  OutputArgumentSpecifications=boolean(true), boolean(true), boolean(true)
  IsPos : Outport
  IsPosZone : Outport  Port=2
  IsPosAlready : Outport  Port=3
  wires:
  Delta/1 -> XXStIsPos_Get/4
  Tolr/1 -> XXStIsPos_Get/5
  PosV/1 -> XXStIsPos_Get/1
  XXStIsPos_Get/2 -> IsPosZone/1
  Pos/1 -> XXStIsPos_Get/2
  XXStIsPos_Get/1 -> IsPos/1
  CalibArray/1 -> XXStIsPos_Get/3
  XXStIsPos_Get/3 -> IsPosAlready/1

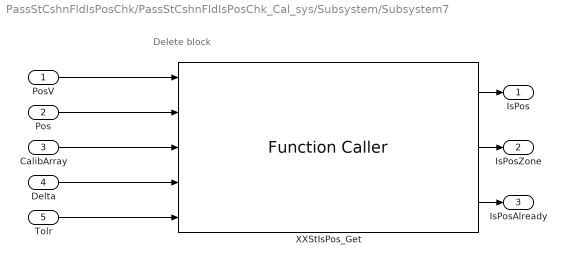
== system PassStCshnFldIsPosChk/PassStCshnFldIsPosChk_Cal_sys/Subsystem/Subsystem7 ==
  note: Delete block
  PosV : Inport
  Pos : Inport  Port=2
  CalibArray : Inport  Port=3
  Delta : Inport  Port=4
  Tolr : Inport  Port=5
  XXStIsPos_Get : FunctionCaller  FunctionPrototype=[IsPos,IsPosZone,IsPosAlready] = XXStIsPos_Get(PosV,Pos,CalibArray,Delta,Tolr)  InputArgumentSpecifications=boolean(true), uint16(1), uint16([1;1;1]), uint16(1), uint16(1)  OutputArgumentSpecifications=boolean(true), boolean(true), boolean(true)
  IsPos : Outport
  IsPosZone : Outport  Port=2
  IsPosAlready : Outport  Port=3
  wires:
  XXStIsPos_Get/3 -> IsPosAlready/1
  CalibArray/1 -> XXStIsPos_Get/3
  XXStIsPos_Get/1 -> IsPos/1
  Pos/1 -> XXStIsPos_Get/2
  XXStIsPos_Get/2 -> IsPosZone/1
  PosV/1 -> XXStIsPos_Get/1
  Tolr/1 -> XXStIsPos_Get/5
  Delta/1 -> XXStIsPos_Get/4

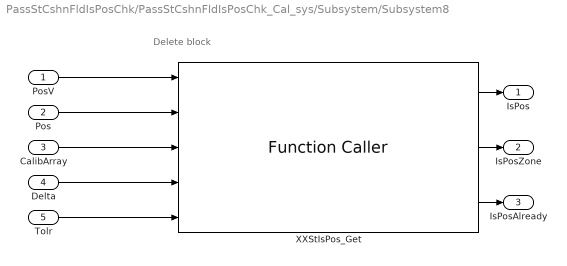
== system PassStCshnFldIsPosChk/PassStCshnFldIsPosChk_Cal_sys/Subsystem/Subsystem8 ==
  note: Delete block
  PosV : Inport
  Pos : Inport  Port=2
  CalibArray : Inport  Port=3
  Delta : Inport  Port=4
  Tolr : Inport  Port=5
  XXStIsPos_Get : FunctionCaller  FunctionPrototype=[IsPos,IsPosZone,IsPosAlready] = XXStIsPos_Get(PosV,Pos,CalibArray,Delta,Tolr)  InputArgumentSpecifications=boolean(true), uint16(1), uint16([1;1;1]), uint16(1), uint16(1)  OutputArgumentSpecifications=boolean(true), boolean(true), boolean(true)
  IsPos : Outport
  IsPosZone : Outport  Port=2
  IsPosAlready : Outport  Port=3
  wires:
  Delta/1 -> XXStIsPos_Get/4
  Tolr/1 -> XXStIsPos_Get/5
  PosV/1 -> XXStIsPos_Get/1
  XXStIsPos_Get/2 -> IsPosZone/1
  Pos/1 -> XXStIsPos_Get/2
  XXStIsPos_Get/1 -> IsPos/1
  CalibArray/1 -> XXStIsPos_Get/3
  XXStIsPos_Get/3 -> IsPosAlready/1
